simulink model "gm_pmsm_decoder_slrt"  (R2020b)
settings: Solver=FixedStepDiscrete  StartTime=0.0  StopTime=20  FixedStep=Ts  RelTol=1e-3
PostLoadFcn:
  | try
  | cell = struct2cell(dir(fullfile(speedgoatroot_hdlb, 'hdlsrc', 'pwm', '*.vhd')));
  | addSourceFiles = strjoin(fullfile(cell(2,:),cell(1,:)), ';');
  | hdlset_param('pwm_example_hdlc/DUT PWM and CAP', 'IPCoreAdditionalFiles', addSourceFiles);
  | end
InitFcn:
  | Ts=50e-6;     % Simulation time step
  | kp = 1e6;   % Proportional gain
  | ki =1e2;   % Integral gain
  | fsw = 5e3;     % Switching frequency
  | Vdc = 400;     % Inverter DC supply voltage
  | Rs = 0.1;     % Stator resistance
  | Ld = 2e-3;   % Inductance (d axis)
  | Lq = 2e-3;   % Inductance (q axis)
  | PM = 0.28;        % Flux linkage
  | N = 1;               % Pole pairs
undefined symbols (not defined in the file): Copy_of_gm_pmsm_fpga_pcie_slrt, DiscIntNeverNeededParam, FPGA, IO334
libraries: speedgoatlib_hdlCoder_IO3xx x19, powerlib x9, powerlib_meascontrol x4, eeGeneralControl x3, quadrature_cpulib x2, mcbcontrolslib x1, slrealtimeutilitieslib x1, pwm_cpulib x1, mcbplantlib x1
settings Model: ModifiedByFormat=Speedgoat GmbH  SimulationMode=external  Creator=Speedgoat GmbH  LastModifiedBy=Speedgoat GmbH
settings SolverCC: ConcurrentTasks=on  PositivePriorityOrder=on
settings DataIOCC: LimitDataPoints=on  SaveFormat=Array  ReturnWorkspaceOutputs=off
settings OptimizationCC: BlockReduction=off  ConditionallyExecuteInputs=off  DefaultParameterBehavior=Inlined  OptimizeBlockIOStorage=off
settings DebuggingCC: AlgebraicLoopMsg=error  UnderspecifiedInitializationDetection=Classic  MergeDetectMultiDrivingBlocksExec=none  SolverPrmCheckMsg=warning  InheritedTsInSrcMsg=none  SingleTaskRateTransMsg=error  TasksWithSamePriorityMsg=none  ParameterPrecisionLossMsg=none  PregeneratedLibrarySubsystemCodeDiagnostic=none  SFUnexpectedBacktrackingDiag=warning  SFNoUnconditionalDefaultTransitionDiag=warning  SFExecutionAtInitializationDiag=none  ArithmeticOperatorsInVariantConditions=warning
settings HardwareCC: ProdBitPerLong=64  ProdLongLongMode=on  ProdHWDeviceType=Intel->x86-64 (Linux 64)  TargetBitPerPointer=64  TargetBitPerSizeT=64  TargetBitPerPtrDiffT=64  TargetLongLongMode=on  TargetIntDivRoundTo=Zero  TargetEndianess=LittleEndian  TargetWordSize=64  TargetHWDeviceType=Custom Processor->MATLAB Host Computer
settings ModelReferenceCC: PropagateSignalLabelsOutOfModel=off
settings SFSimCC: SimUseLocalCustomCode=off  CustomCodeUndefinedFunction=UseInterfaceOnly
settings RTWCC: Description=Simulink Real-Time  SystemTargetFile=slrealtime.tlc  TemplateMakefile=slrealtime_default_tmf  RTWUseLocalCustomCode=off  Toolchain=Simulink Real-Time Toolchain  BuildConfiguration=Faster Runs  CodeExecutionProfiling=on  TargetLang=C++
settings CodeAppCC: StateflowObjectComments=on
settings ConfigComp: CovMetricSettings=dw  CovSaveCumulativeToWorkspaceVar=on  CovSaveSingleToWorkspaceVar=on  CovExternalEMLEnable=off

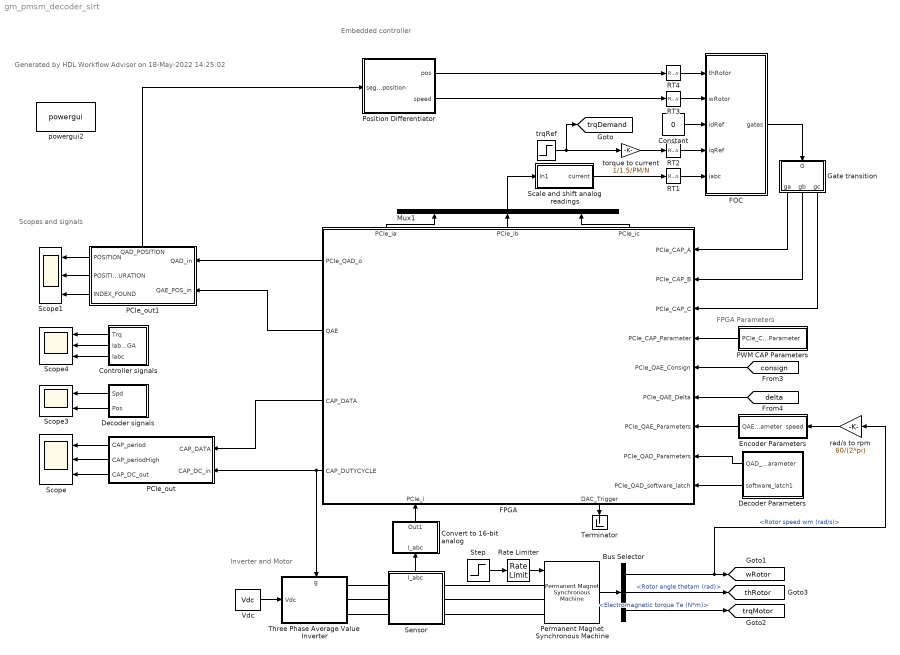
== system gm_pmsm_decoder_slrt ==
  note: Inverter and Motor
  note: FPGA Parameters
  note: Embedded controller
  note: Scopes and signals
  note: Generated by HDL Workflow Advisor on 18-May-2022 14:25:02
  Bus Selector : BusSelector  OutputSignals=Rotor speed wm (rad/s),Rotor angle thetam (rad),Electromagnetic torque Te (N*m)
  Constant : Constant  Value=0  SampleTime=-1
  Controller signals : Subsystem
  Convert to 16-bit analog : Subsystem
  Decoder Parameters : Subsystem
  Decoder signals : Subsystem
  Encoder Parameters : Subsystem
  FOC : Subsystem
  FPGA : Subsystem  mask(Speedgoat IO334-325k Interface Block){module_id=1, slot=-1, ts=-1, FpgaFreq=100}
      mask prompts: module_id "FPGA Module Identifier:"; slot "PCI slot (-1: autosearch):"; ts "Sample time:"; FpgaFreq "FPGA Frequency [MHz]"
      mask help: Simulink Real-Time Interface Block for Speedgoat IO334-325k.
      mask init:
      | hdlslrt.backend.mfpgaparameters;
      settings: PortSchema="{\"entries\":[{\"content\":{\"sides\":[{\"content\":{\"connectorIds\":[\"Out5\",\"Out6\",\"Out7\",\"Out8\"]},\"type\":\"ConnectorPlacement.EquallySpacedRectSide\",\"uuid\":\"34ddc533-e92e-4f84-ab54-56ee31c34ed5\"},{\"content\":{\"connectorIds\":[\"In2\",\"In3\",\"In4\",\"In5\",\"In6\",\"In7\",\"In8\",\"In9\",\"In10\"],\"side\":\"RIGHT\"},\"type\":\"ConnectorPlacement.EquallySpacedRectSide\",\"uuid\":\"fc43732f-8b85-47c9-af73-b87840a05fb5\"},{\"content\":{\"connectorIds\":[\"Out2\",\"Out3\",\"Out4\"],\"side\":\"TOP\"},\"type\":\"ConnectorPlacement.EquallySpacedRectSide\",\"uuid\":\"bf663b9c-33b6-4726-afdb-56df835214b8\"},{\"content\":{\"connectorIds\":[\"In1\",\"Out1\"],\"side\":\"BOTTOM\"},\"type\":\"ConnectorPlacement.EquallySpacedRectSide\",\"uuid\":\"04fbffa8-14ef-4425-a219-a420a37a7cbf\"},{\"content\":{\"connectorIds\":[],\"side\":\"HIDDEN\"},\"type\":\"ConnectorPlacement.EquallySpacedRectSide\",\"uuid\":\"ed9b2637-afe7-435a-b994-99eac90c9c32\"}]},\"type\":\"ConnectorPlacement.EquallySpacedConnector\",\"uuid\":\"b4b9272a-3f4d-4e79-a573-4a3ad4933ba9\"}],\"packageUris\":[\"http://schema.mathworks.com/mf0/Connector/R2020b\"],\"version\":\"1.0\"}"
      mask Help: eval('speedgoatdoc_hdlc')
      mask Display:
      | SetupBlkPath = find_system(gcb, 'LookUnderMasks', 'all', 'FollowLinks', 'on', 'regexp', 'on', 'Name', 'IO3(\d|x){2}\s+Setup' );
      | SetupBlkPath = SetupBlkPath{1};
      | TS = get_param(SetupBlkPath,'timestamp_mcs');
      | disp(sprintf('Speedgoat IO334-325k\nFPGA I/O Module\n\nTimestamp\n%s\n\nReference Design\nVersion 2.1\n\nMatlab R2020b\n\nPCIe Link Width: X4\nRear Plugin: -21\nAurora Mode: None\nAurora Byteswap: true\n', TS))
  Gate transition : Subsystem
  Mux1 : Mux  Inputs=3
  PCIe_out : Subsystem
  PCIe_out1 : Subsystem
      settings: PortSchema="{\"entries\":[{\"content\":{\"sides\":[{\"content\":{\"connectorIds\":[\"In1\",\"In2\"]},\"type\":\"ConnectorPlacement.EquallySpacedRectSide\",\"uuid\":\"af69b108-ebc1-4eba-857b-579d7c2071b1\"},{\"content\":{\"connectorIds\":[\"Out1\",\"Out2\",\"Out3\"],\"side\":\"RIGHT\"},\"type\":\"ConnectorPlacement.EquallySpacedRectSide\",\"uuid\":\"109121c9-5293-4b78-b0df-8505743611a0\"},{\"content\":{\"connectorIds\":[\"Out4\"],\"side\":\"TOP\"},\"type\":\"ConnectorPlacement.EquallySpacedRectSide\",\"uuid\":\"7680958f-0bbc-4169-a54e-ff3c19fd2e64\"},{\"content\":{\"connectorIds\":[],\"side\":\"HIDDEN\"},\"type\":\"ConnectorPlacement.EquallySpacedRectSide\",\"uuid\":\"af8ad87e-ac41-49e8-9442-a6b24975ced8\"}]},\"type\":\"ConnectorPlacement.EquallySpacedConnector\",\"uuid\":\"27b07649-0e95-47d8-9bc5-7790ead06fb5\"}],\"packageUris\":[\"http://schema.mathworks.com/mf0/Connector/R2020b\"],\"version\":\"1.0\"}"
  PWM CAP Parameters : Subsystem
  Permanent Magnet Synchronous Machine : powerlib/Machines/Permanent Magnet Synchronous Machine  NbPhases=3  FluxDistribution=Sinusoidal  RotorType=Salient-pole  MechanicalLoad=Speed w  PresetModel=No  ShowDetailedParameters=on  MeasurementBus=off  Resistance=Rs  Inductance=8.5e-3  dqInductances=[Ld Lq]  La=0.000395  MachineConstant=Flux linkage established by magnets (V.s)  Flux=PM  VoltageCst=50.7864  TorqueCst=0.42  Flat=120  Mechanical=[0.0027 0.0004924 1 0]  PolePairs=N  InitialConditions=[0,0, 0,0]  InitialConditions5ph=[0 0 0 0 0 0]  RefAngle=Aligned with phase A axis (original Park)  IterativeDiscreteModel=Trapezoidal non iterative  TsBlock=-1  TsPowergui=0
  Position Differentiator : Subsystem
  RT{1..4} (4 alike) : RateTransition  OutPortSampleTimeOpt=Inherit  OutPortSampleTime=Ts
  Rate Limiter : RateLimiter  RisingSlewLimit=100/60*2*pi  SampleTimeMode=inherited
  Scale and shift analog readings : Subsystem
  Scope : Scope  NumInputPorts=3
  Scope1 : Scope  NumInputPorts=3
  Scope3 : Scope  NumInputPorts=2
  Scope4 : Scope  NumInputPorts=3
  Sensor : Subsystem
      settings: PortSchema="{\"entries\":[{\"content\":{\"sides\":[{\"content\":{\"connectorIds\":[\"LConn1\",\"LConn2\",\"LConn3\"]},\"type\":\"ConnectorPlacement.EquallySpacedRectSide\",\"uuid\":\"d3673cf9-f798-4f95-832a-0ee38b3b4235\"},{\"content\":{\"connectorIds\":[\"RConn1\",\"RConn2\",\"RConn3\"],\"side\":\"RIGHT\"},\"type\":\"ConnectorPlacement.EquallySpacedRectSide\",\"uuid\":\"f1c3e6c7-7356-4e8b-bcca-414f2c82a0be\"},{\"content\":{\"connectorIds\":[\"Out1\"],\"side\":\"TOP\"},\"type\":\"ConnectorPlacement.EquallySpacedRectSide\",\"uuid\":\"10e31bf8-a182-46d8-beca-1ec9bb9081e0\"},{\"content\":{\"connectorIds\":[],\"side\":\"HIDDEN\"},\"type\":\"ConnectorPlacement.EquallySpacedRectSide\",\"uuid\":\"21150a95-24d3-4ba1-92b8-5619804d049c\"}]},\"type\":\"ConnectorPlacement.EquallySpacedConnector\",\"uuid\":\"db0d9e3c-2d98-4024-a8e1-7fc9e86b9a02\"}],\"packageUris\":[\"http://schema.mathworks.com/mf0/Connector/R2020b\"],\"version\":\"1.0\"}"
  Step : Step  Time=0.01  After=500/60*2*pi  SampleTime=0
  Terminator : Terminator
  Three Phase Average Value Inverter : Subsystem
      settings: PortSchema="{\"entries\":[{\"content\":{\"sides\":[{\"content\":{\"connectorIds\":[\"In1\"]},\"type\":\"ConnectorPlacement.EquallySpacedRectSide\",\"uuid\":\"bfacb710-2d3a-4e7b-9063-25c8b87226b9\"},{\"content\":{\"connectorIds\":[\"RConn1\",\"RConn2\",\"RConn3\"],\"side\":\"RIGHT\"},\"type\":\"ConnectorPlacement.EquallySpacedRectSide\",\"uuid\":\"a8d38f79-eb95-4afe-ba2f-2842c1cba801\"},{\"content\":{\"connectorIds\":[\"In2\"],\"side\":\"TOP\"},\"type\":\"ConnectorPlacement.EquallySpacedRectSide\",\"uuid\":\"291d9d52-08e6-4456-8afe-095013b7df64\"},{\"content\":{\"connectorIds\":[],\"side\":\"HIDDEN\"},\"type\":\"ConnectorPlacement.EquallySpacedRectSide\",\"uuid\":\"61aa80b0-9b99-474b-ab67-e014373e5595\"}]},\"type\":\"ConnectorPlacement.EquallySpacedConnector\",\"uuid\":\"1232c420-125a-43af-99e1-be04cd6c95a4\"}],\"packageUris\":[\"http://schema.mathworks.com/mf0/Connector/R2020b\"],\"version\":\"1.0\"}"
  Vdc : Constant  Value=Vdc  SampleTime=Ts
  powergui2 : powerlib/powergui  Priority=1  SimulationMode=Discrete  SampleTime=Ts  frequency=60  Iterations=50  frequencyindice=0  Pbase=100e6  ErrMax=1e-4  UnitsV=kV  UnitsW=MW  buscounter=0  FunctionMessages=off  echomessages=off  EnableUseOfTLC=off  CurrentSourceSwitches=off  DisableSnubberDevices=off  DisableRonSwitches=off  DisableVfSwitches=off  DisplayEquations=off  AutomaticDiscreteSolvers=off  SolverType=Tustin/Backward Euler (TBE)  Interpol=off  ExternalGateDelay=off  methode=off  Ts=100  x0status=blocks  SPID=on  SwTol=0  HookPort=off  NonlinearTolerance=1e-4  nMaxIteration=100  ContinueOnMaxIteration=off  RestoreLinks=warning  ResistiveCurrentMeasurement=off  Frange=[0:2:500]  Ylog=off  Xlog=on  ShowGrid=off  save=off  variable=ZData  structure=0  ZoomFFT=off  StartTime=0.0  cycles=1  DisplayStyle=1  fundamental=60  FreqAxis=off  MaxFrequency=1000  frequencyindicesteady=1  RmsSteady=1  display=off
  rad/s to rpm : Gain  Gain=60/(2*pi)
  torque to current : Gain  Gain=1/1.5/PM/N  SaturateOnIntegerOverflow=on  OutDataTypeStr=Inherit: Same as input  ParamDataTypeStr=Inherit: Same as input
  trqRef : Step  Time=0.3  After=300  SampleTime=Ts
  tag scope: thRotor=global, trqDemand=global, trqMotor=global, wRotor=global
  wires:
  Convert to 16-bit analog/1(Out1) -> FPGA/1(PCIe_i)
  Decoder Parameters/2(software_latch1) -> FPGA/10(PCIe_QAD_software_latch)
  Decoder Parameters/1(QAD_parameter) -> FPGA/9(PCIe_QAD_Parameters)
  FPGA/5(PCIe_QAD_o) -> PCIe_out1/1(QAD_in)
  PCIe_out1/2(POSITION_DURATION) -> Scope1/2
  PCIe_out1/3(INDEX_FOUND) -> Scope1/3
  PCIe_out1/1(POSITION) -> Scope1/1
  RT4/1 -> FOC/1(thRotor)
  Controller signals/3(Iabc) -> Scope4/3
  Controller signals/2(Iabc_FPGA) -> Scope4/2
  Controller signals/1(Trq) -> Scope4/1
  Rate Limiter/1 -> Permanent Magnet Synchronous Machine/1
  Vdc/1 -> Three Phase Average Value Inverter/1(Vdc)
  Bus Selector/2 -> [thRotor]  "<Rotor angle thetam (rad)>"
  FPGA/8(CAP_DUTYCYCLE) -> Three Phase Average Value Inverter/2(g), PCIe_out/2(CAP_DC_in)
  Sensor/1(I_abc) -> Convert to 16-bit analog/1(I_abc)
  Bus Selector/1 -> [wRotor], rad/s to rpm/1  "<Rotor speed wm (rad/s)>"
  Permanent Magnet Synchronous Machine/1 -> Bus Selector/1
  Bus Selector/3 -> [trqMotor]  "<Electromagnetic torque Te (N*m)>"
  FOC/1(gates) -> Gate transition/1(G)
  Constant/1 -> FOC/3(idRef)
  torque to current/1 -> RT2/1
  PCIe_out/3(CAP_DC_out) -> Scope/3
  PCIe_out/2(CAP_periodHigh) -> Scope/2
  PCIe_out/1(CAP_period) -> Scope/1
  Encoder Parameters/1(QAE_parameter) -> FPGA/8(PCIe_QAE_Parameters)
  PWM CAP Parameters/1(PCIe_CAP_Parameter) -> FPGA/5(PCIe_CAP_Parameter)
  FPGA/7(CAP_DATA) -> PCIe_out/1(CAP_DATA)
  rad/s to rpm/1 -> Encoder Parameters/1(speed)
  FPGA/6(QAE) -> PCIe_out1/2(QAE_POS_in)
  RT3/1 -> FOC/2(wRotor)
  RT2/1 -> FOC/4(iqRef)
  RT1/1 -> FOC/5(iabc)
  trqRef/1 -> torque to current/1, [trqDemand]
  FPGA/3(PCIe_ib) -> Mux1/2
  FPGA/2(PCIe_ia) -> Mux1/1
  FPGA/4(PCIe_ic) -> Mux1/3
  FPGA/1(DAC_Trigger) -> Terminator/1
  Decoder signals/1(Spd) -> Scope3/1
  Decoder signals/2(Pos) -> Scope3/2
  [delta] -> FPGA/7(PCIe_QAE_Delta)
  [consign] -> FPGA/6(PCIe_QAE_Consign)
  Gate transition/1(ga) -> FPGA/2(PCIe_CAP_A)
  Gate transition/2(gb) -> FPGA/3(PCIe_CAP_B)
  Gate transition/3(gc) -> FPGA/4(PCIe_CAP_C)
  Mux1/1 -> Scale and shift analog readings/1(In1)
  Scale and shift analog readings/1(current) -> RT1/1
  Step/1 -> Rate Limiter/1
  PCIe_out1/4(QAD_POSITION) -> Position Differentiator/1(segment position)
  Position Differentiator/1(pos) -> RT4/1
  Position Differentiator/2(speed) -> RT3/1
  connections:
  Permanent Magnet Synchronous Machine/LConn2 -- Sensor/RConn2
  Permanent Magnet Synchronous Machine/LConn3 -- Sensor/RConn3
  Sensor/LConn3 -- Three Phase Average Value Inverter/RConn3
  Sensor/LConn1 -- Three Phase Average Value Inverter/RConn1
  Sensor/LConn2 -- Three Phase Average Value Inverter/RConn2
  Permanent Magnet Synchronous Machine/LConn1 -- Sensor/RConn1

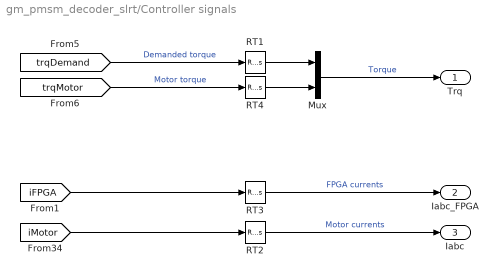
== system gm_pmsm_decoder_slrt/Controller signals ==
  Mux : Mux  Inputs=2
  RT{1..4} (4 alike) : RateTransition  OutPortSampleTime=Ts
  Trq : Outport  VectorParamsAs1DForOutWhenUnconnected=off
  Iabc_FPGA : Outport  Port=2  VectorParamsAs1DForOutWhenUnconnected=off
  Iabc : Outport  Port=3  VectorParamsAs1DForOutWhenUnconnected=off
  wires:
  [trqDemand] -> RT1/1  "Demanded torque"
  RT1/1 -> Mux/1
  RT3/1 -> Iabc_FPGA/1  "FPGA currents"
  [iMotor] -> RT2/1
  RT2/1 -> Iabc/1  "Motor currents"
  [iFPGA] -> RT3/1
  Mux/1 -> Trq/1  "Torque"
  [trqMotor] -> RT4/1  "Motor torque"
  RT4/1 -> Mux/2

== system gm_pmsm_decoder_slrt/Convert to 16-bit analog ==
  I_abc : Inport
  1-D Lookup Table : Lookup_n-D  NumberOfTableDimensions=1  BreakpointsForDimension1=[-2^15, 2^15-1]  Table=[0, 3.3/10*(2^15-1)]  ExtrapMethod=Clip  InternalRulePriority=Speed  RndMeth=Simplest  InputSameDT=on
  Data Type Conversion : DataTypeConversion  OutDataTypeStr=int16
  Gain : Gain  Gain=2^3
  Out1 : Outport
  wires:
  Data Type Conversion/1 -> Out1/1
  1-D Lookup Table/1 -> Data Type Conversion/1
  I_abc/1 -> Gain/1
  Gain/1 -> 1-D Lookup Table/1

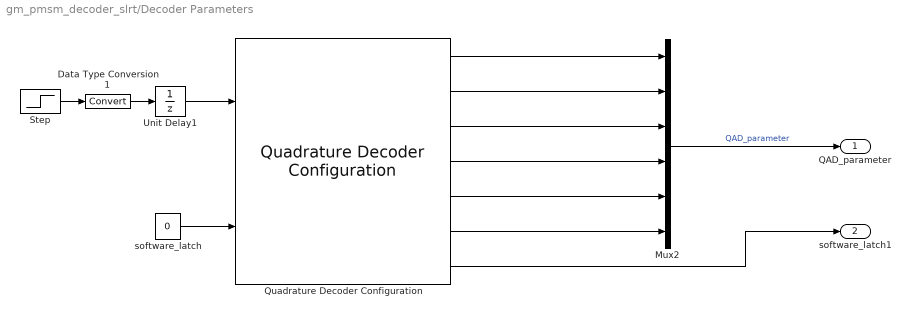
== system gm_pmsm_decoder_slrt/Decoder Parameters ==
  Data Type Conversion1 : DataTypeConversion
  Mux2 : Mux  Inputs=6
  Quadrature Decoder Configuration : quadrature_cpulib/Quadrature Decoder Configuration  FPGA_freq=100e6  n_channels=1  samplingMode=2x  indexControlMode=Reset on index  latchMode=Continuous  lowerLimit=0  upperLimit=512
      settings: SourceProductName=Simulink Real-Time: Speedgoat HDL Blockset
  Step : Step  Time=0.002
  Unit Delay1 : UnitDelay  SampleTime=-1  HasFrameUpgradeWarning=on
  software_latch : Constant  Value=0  SampleTime=-1
  QAD_parameter : Outport
  software_latch1 : Outport  Port=2
  wires:
  Quadrature Decoder Configuration/7 -> software_latch1/1
  Mux2/1 -> QAD_parameter/1  "QAD_parameter"
  software_latch/1 -> Quadrature Decoder Configuration/2
  Quadrature Decoder Configuration/1 -> Mux2/1
  Quadrature Decoder Configuration/6 -> Mux2/6
  Quadrature Decoder Configuration/4 -> Mux2/4
  Quadrature Decoder Configuration/3 -> Mux2/3
  Data Type Conversion1/1 -> Unit Delay1/1
  Quadrature Decoder Configuration/5 -> Mux2/5
  Step/1 -> Data Type Conversion1/1
  Unit Delay1/1 -> Quadrature Decoder Configuration/1
  Quadrature Decoder Configuration/2 -> Mux2/2

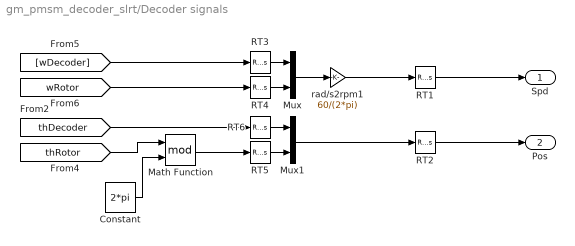
== system gm_pmsm_decoder_slrt/Decoder signals ==
  Constant : Constant  Value=2*pi  SampleTime=-1
  Math Function : Math  Operator=mod  SaturateOnIntegerOverflow=on
  Mux : Mux  Inputs=2
  Mux1 : Mux  Inputs=2
  RT{1..6} (6 alike) : RateTransition  OutPortSampleTime=Ts
  rad/s2rpm1 : Gain  Gain=60/(2*pi)
  Spd : Outport  VectorParamsAs1DForOutWhenUnconnected=off
  Pos : Outport  Port=2  VectorParamsAs1DForOutWhenUnconnected=off
  wires:
  [wDecoder] -> RT3/1
  Mux/1 -> rad/s2rpm1/1
  Mux1/1 -> RT2/1
  [wRotor] -> RT4/1
  RT1/1 -> Spd/1
  RT2/1 -> Pos/1
  RT4/1 -> Mux/2
  RT5/1 -> Mux1/2
  rad/s2rpm1/1 -> RT1/1
  RT3/1 -> Mux/1
  RT6/1 -> Mux1/1
  [thDecoder] -> RT6/1
  Constant/1 -> Math Function/2
  [thRotor] -> Math Function/1
  Math Function/1 -> RT5/1

== system gm_pmsm_decoder_slrt/Encoder Parameters ==
  speed : Inport
  Mux2 : Mux  Inputs=7
  Quadrature Encoder Configuration : quadrature_cpulib/Quadrature Encoder Configuration  fpgaFreq=100e6  n_channels=1  numSeg=[512]  phaseAngle=90  initPos=[0]  freeWheel=on
      settings: SourceProductName=Simulink Real-Time: Speedgoat HDL Blockset
  Step : Step  Time=0.002
  position : Constant  Value=8  SampleTime=-1
  QAE_parameter : Outport
  tag scope: consign=global, delta=global
  wires:
  speed/1 -> Quadrature Encoder Configuration/3
  Quadrature Encoder Configuration/8 -> [consign]
  Step/1 -> Quadrature Encoder Configuration/1
  Quadrature Encoder Configuration/7 -> Mux2/7
  Quadrature Encoder Configuration/4 -> Mux2/4
  Quadrature Encoder Configuration/2 -> Mux2/2
  position/1 -> Quadrature Encoder Configuration/2
  Mux2/1 -> QAE_parameter/1  "QAE_parameter"
  Quadrature Encoder Configuration/6 -> Mux2/6
  Quadrature Encoder Configuration/5 -> Mux2/5
  Quadrature Encoder Configuration/1 -> Mux2/1  "position"
  Quadrature Encoder Configuration/9 -> [delta]
  Quadrature Encoder Configuration/3 -> Mux2/3

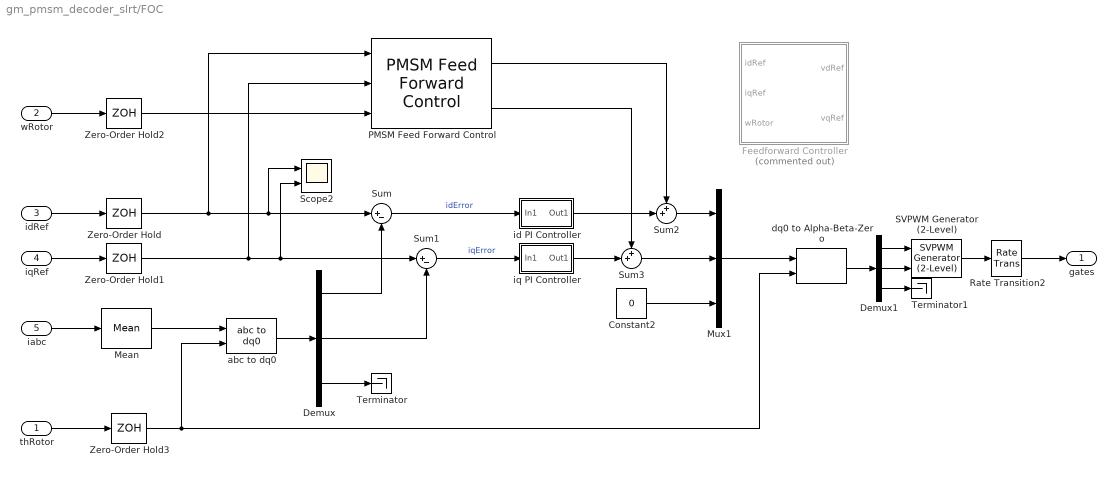
== system gm_pmsm_decoder_slrt/FOC ==
  thRotor : Inport
  wRotor : Inport  Port=2
  idRef : Inport  Port=3
  iqRef : Inport  Port=4
  iabc : Inport  Port=5
  Constant2 : Constant  Value=0  SampleTime=-1
  Demux : Demux  Outputs=3
  Demux1 : Demux  Outputs=3
  Feedforward Controller : Subsystem  Commented=on
  Mean : powerlib_meascontrol/Measurements/Mean  Freq=fsw  Vinit=0  Ts=Ts
  Mux1 : Mux  Inputs=3
  PMSM Feed Forward Control : mcbcontrolslib/PMSM Feed Forward Control  polePairs=N  Ld=Ld  Lq=Lq  FluxPM=PM  V_dc=Vdc/sqrt(3)  Units=SI Units  V_base=24/sqrt(3)  I_base=19.3  N_base=4107
      settings: SourceProductBaseCode=MT
  Rate Transition2 : RateTransition
  SVPWM Generator (2-Level) : powerlib_meascontrol/Pulse & Signal Generators/SVPWM Generator (2-Level)  InputType=alpha-beta components  SwitchingPattern=Pattern #1  Fc=fsw  ParUref=[0.8 -30 50]  Ts=Ts
      settings: SourceProductBaseCode=PS
  Scope2 : Scope  NumInputPorts=2
  Sum : Sum  Inputs=|+-
  Sum1 : Sum  Inputs=|+-
  Sum2 : Sum  Inputs=++|
  Sum3 : Sum  Inputs=++|
  Terminator : Terminator
  Terminator1 : Terminator
  Zero-Order Hold{,1..3} (4 alike) : ZeroOrderHold  SampleTime=-1
  abc to dq0 : powerlib_meascontrol/Transformations/abc to dq0  Alignment=Aligned with phase A axis
  dq0 to Alpha-Beta-Zero : powerlib_meascontrol/Transformations/dq0 to Alpha-Beta-Zero  Alignment=Aligned with phase A axis
      settings: SourceProductBaseCode=PS
  id PI Controller : Subsystem
  iq PI Controller : Subsystem
  gates : Outport  VectorParamsAs1DForOutWhenUnconnected=off
  wires:
  Zero-Order Hold3/1 -> dq0 to Alpha-Beta-Zero/2, abc to dq0/2
  Zero-Order Hold2/1 -> PMSM Feed Forward Control/3
  iqRef/1 -> Zero-Order Hold1/1
  idRef/1 -> Zero-Order Hold/1
  PMSM Feed Forward Control/2 -> Sum3/1
  PMSM Feed Forward Control/1 -> Sum2/1
  Constant2/1 -> Mux1/3
  Demux/1 -> Sum/2
  dq0 to Alpha-Beta-Zero/1 -> Demux1/1
  Demux1/2 -> SVPWM Generator (2-Level)/2
  SVPWM Generator (2-Level)/1 -> Rate Transition2/1
  id PI Controller/1(Out1) -> Sum2/2
  Sum2/1 -> Mux1/1
  Sum3/1 -> Mux1/2
  Demux/2 -> Sum1/2
  Sum1/1 -> iq PI Controller/1(In1)  "iqError"
  iabc/1 -> Mean/1
  Demux1/3 -> Terminator1/1
  Mux1/1 -> dq0 to Alpha-Beta-Zero/1
  Mean/1 -> abc to dq0/1
  wRotor/1 -> Zero-Order Hold2/1
  thRotor/1 -> Zero-Order Hold3/1
  Rate Transition2/1 -> gates/1
  Zero-Order Hold1/1 -> Scope2/2, Sum1/1, PMSM Feed Forward Control/2
  abc to dq0/1 -> Demux/1
  Sum/1 -> id PI Controller/1(In1)  "idError"
  Demux1/1 -> SVPWM Generator (2-Level)/1
  Zero-Order Hold/1 -> Sum/1, Scope2/1, PMSM Feed Forward Control/1
  iq PI Controller/1(Out1) -> Sum3/2
  Demux/3 -> Terminator/1

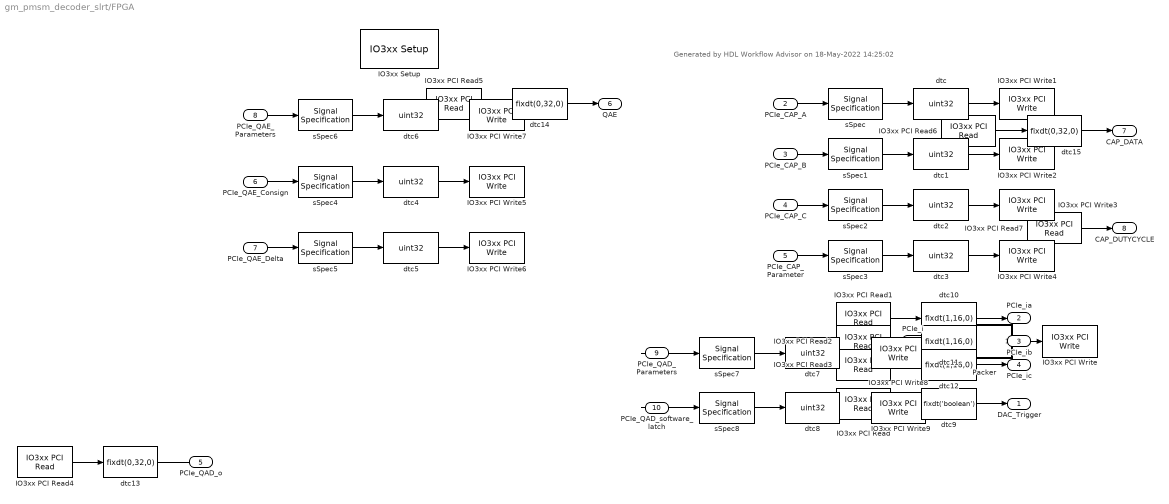
== system gm_pmsm_decoder_slrt/FPGA ==
  note: Generated by HDL Workflow Advisor on 18-May-2022 14:25:02
  PCIe_i : Inport  OutDataTypeStr=int16
  PCIe_CAP_A : Inport  Port=2
  PCIe_CAP_B : Inport  Port=3
  PCIe_CAP_C : Inport  Port=4
  PCIe_CAP_Parameter : Inport  Port=5
  PCIe_QAE_Consign : Inport  Port=6
  PCIe_QAE_Delta : Inport  Port=7
  PCIe_QAE_Parameters : Inport  Port=8
  PCIe_QAD_Parameters : Inport  Port=9
  PCIe_QAD_software_latch : Inport  Port=10
  IO3xx PCI Read : speedgoatlib_hdlCoder_IO3xx/IO3xx PCI Read  device_id=1  module_id=module_id  board_type=IO334-325k  port_name=DAC_Trigger  port_offset=hex2dec('134')  port_type=uint32  port_dim=1  strobe=0  sample_time=ts
  IO3xx PCI Read1 : speedgoatlib_hdlCoder_IO3xx/IO3xx PCI Read  device_id=1  module_id=module_id  board_type=IO334-325k  port_name=PCIe_ia  port_offset=hex2dec('138')  port_type=uint32  port_dim=1  strobe=0  sample_time=ts
  IO3xx PCI Read2 : speedgoatlib_hdlCoder_IO3xx/IO3xx PCI Read  device_id=1  module_id=module_id  board_type=IO334-325k  port_name=PCIe_ib  port_offset=hex2dec('13C')  port_type=uint32  port_dim=1  strobe=0  sample_time=ts
  IO3xx PCI Read3 : speedgoatlib_hdlCoder_IO3xx/IO3xx PCI Read  device_id=1  module_id=module_id  board_type=IO334-325k  port_name=PCIe_ic  port_offset=hex2dec('144')  port_type=uint32  port_dim=1  strobe=0  sample_time=ts
  IO3xx PCI Read4 : speedgoatlib_hdlCoder_IO3xx/IO3xx PCI Read  device_id=1  module_id=module_id  board_type=IO334-325k  port_name=PCIe_QAD_o  port_offset=hex2dec('1D0')  port_type=uint32  port_dim=4  strobe=hex2dec('1E0')  sample_time=ts
  IO3xx PCI Read5 : speedgoatlib_hdlCoder_IO3xx/IO3xx PCI Read  device_id=1  module_id=module_id  board_type=IO334-325k  port_name=QAE  port_offset=hex2dec('150')  port_type=uint32  port_dim=1  strobe=0  sample_time=ts
  IO3xx PCI Read6 : speedgoatlib_hdlCoder_IO3xx/IO3xx PCI Read  device_id=1  module_id=module_id  board_type=IO334-325k  port_name=CAP_DATA  port_offset=hex2dec('200')  port_type=uint32  port_dim=18  strobe=hex2dec('280')  sample_time=ts
  IO3xx PCI Read7 : speedgoatlib_hdlCoder_IO3xx/IO3xx PCI Read  device_id=1  module_id=module_id  board_type=IO334-325k  port_name=CAP_DUTYCYCLE  port_offset=hex2dec('290')  port_type=single  port_dim=3  strobe=hex2dec('2A0')  sample_time=ts
  IO3xx PCI Write : speedgoatlib_hdlCoder_IO3xx/IO3xx PCI Write  device_id=1  module_id=module_id  board_type=IO334-325k  port_name=PCIe_i  port_offset=hex2dec('100')  port_type=uint32  port_dim=2  strobe=hex2dec('108')  sample_time=ts
  IO3xx PCI Write1 : speedgoatlib_hdlCoder_IO3xx/IO3xx PCI Write  device_id=1  module_id=module_id  board_type=IO334-325k  port_name=PCIe_CAP_A  port_offset=hex2dec('10C')  port_type=uint32  port_dim=1  strobe=0  sample_time=ts
  IO3xx PCI Write2 : speedgoatlib_hdlCoder_IO3xx/IO3xx PCI Write  device_id=1  module_id=module_id  board_type=IO334-325k  port_name=PCIe_CAP_B  port_offset=hex2dec('110')  port_type=uint32  port_dim=1  strobe=0  sample_time=ts
  IO3xx PCI Write3 : speedgoatlib_hdlCoder_IO3xx/IO3xx PCI Write  device_id=1  module_id=module_id  board_type=IO334-325k  port_name=PCIe_CAP_C  port_offset=hex2dec('114')  port_type=uint32  port_dim=1  strobe=0  sample_time=ts
  IO3xx PCI Write4 : speedgoatlib_hdlCoder_IO3xx/IO3xx PCI Write  device_id=1  module_id=module_id  board_type=IO334-325k  port_name=PCIe_CAP_Parameter  port_offset=hex2dec('120')  port_type=uint32  port_dim=3  strobe=hex2dec('130')  sample_time=ts
  IO3xx PCI Write5 : speedgoatlib_hdlCoder_IO3xx/IO3xx PCI Write  device_id=1  module_id=module_id  board_type=IO334-325k  port_name=PCIe_QAE_Consign  port_offset=hex2dec('140')  port_type=uint32  port_dim=1  strobe=0  sample_time=ts
  IO3xx PCI Write6 : speedgoatlib_hdlCoder_IO3xx/IO3xx PCI Write  device_id=1  module_id=module_id  board_type=IO334-325k  port_name=PCIe_QAE_Delta  port_offset=hex2dec('118')  port_type=uint32  port_dim=1  strobe=0  sample_time=ts
  IO3xx PCI Write7 : speedgoatlib_hdlCoder_IO3xx/IO3xx PCI Write  device_id=1  module_id=module_id  board_type=IO334-325k  port_name=PCIe_QAE_Parameters  port_offset=hex2dec('160')  port_type=uint32  port_dim=7  strobe=hex2dec('180')  sample_time=ts
  IO3xx PCI Write8 : speedgoatlib_hdlCoder_IO3xx/IO3xx PCI Write  device_id=1  module_id=module_id  board_type=IO334-325k  port_name=PCIe_QAD_Parameters  port_offset=hex2dec('1A0')  port_type=uint32  port_dim=6  strobe=hex2dec('1C0')  sample_time=ts
  IO3xx PCI Write9 : speedgoatlib_hdlCoder_IO3xx/IO3xx PCI Write  device_id=1  module_id=module_id  board_type=IO334-325k  port_name=PCIe_QAD_software_latch  port_offset=hex2dec('11C')  port_type=uint32  port_dim=1  strobe=0  sample_time=ts
  IO3xx Setup : speedgoatlib_hdlCoder_IO3xx/IO3xx Setup  mdl_ss_name=Copy_of_gm_pmsm_fpga_pcie_slrt/FPGA  board_type=IO334-325k  fpga_sync_mode=on  reset_mode=on  device_id=1  module_id=module_id  pci_slot=slot  fpga_mat_file=hdl_prj\hdlsrc\Copy_of_gm_pmsm_fpga_pcie_slrt\FPGA.mat  timestamp_mcs=05/18/22 14:10:29  timestamp=2205181323  tsreg=hex2dec('8')  bsf_file=FPGA_2205181323.mcs  mcs=0
  Packer : Subsystem
  dtc{,1..8} (9 alike) : DataTypeConversion  OutDataTypeStr=uint32  ConvertRealWorld=Stored Integer (SI)  RndMeth=Zero
  dtc10 : DataTypeConversion  OutDataTypeStr=fixdt(1,16,0)  ConvertRealWorld=Stored Integer (SI)  RndMeth=Zero
  dtc11 : DataTypeConversion  OutDataTypeStr=fixdt(1,16,0)  ConvertRealWorld=Stored Integer (SI)  RndMeth=Zero
  dtc12 : DataTypeConversion  OutDataTypeStr=fixdt(1,16,0)  ConvertRealWorld=Stored Integer (SI)  RndMeth=Zero
  dtc13 : DataTypeConversion  OutDataTypeStr=fixdt(0,32,0)  ConvertRealWorld=Stored Integer (SI)  RndMeth=Zero
  dtc14 : DataTypeConversion  OutDataTypeStr=fixdt(0,32,0)  ConvertRealWorld=Stored Integer (SI)  RndMeth=Zero
  dtc15 : DataTypeConversion  OutDataTypeStr=fixdt(0,32,0)  ConvertRealWorld=Stored Integer (SI)  RndMeth=Zero
  dtc9 : DataTypeConversion  OutDataTypeStr=fixdt('boolean')  ConvertRealWorld=Stored Integer (SI)  RndMeth=Zero
  sSpec{,1..2,8} (4 alike) : SignalSpecification  OutDataTypeStr=fixdt('boolean')
  sSpec3 : SignalSpecification  OutDataTypeStr=fixdt(0,32,0)
  sSpec4 : SignalSpecification  OutDataTypeStr=fixdt(0,32,0)
  sSpec5 : SignalSpecification  OutDataTypeStr=fixdt(1,32,0)
  sSpec6 : SignalSpecification  OutDataTypeStr=fixdt(0,32,0)
  sSpec7 : SignalSpecification  OutDataTypeStr=fixdt(1,32,0)
  DAC_Trigger : Outport
  PCIe_ia : Outport  Port=2
  PCIe_ib : Outport  Port=3
  PCIe_ic : Outport  Port=4
  PCIe_QAD_o : Outport  Port=5  VectorParamsAs1DForOutWhenUnconnected=off
  QAE : Outport  Port=6
  CAP_DATA : Outport  Port=7
  CAP_DUTYCYCLE : Outport  Port=8
  wires:
  PCIe_i/1 -> Packer/1(unpacked)
  Packer/1(packed) -> IO3xx PCI Write/1
  PCIe_CAP_A/1 -> sSpec/1
  sSpec/1 -> dtc/1
  dtc/1 -> IO3xx PCI Write1/1
  PCIe_CAP_B/1 -> sSpec1/1
  sSpec1/1 -> dtc1/1
  dtc1/1 -> IO3xx PCI Write2/1
  PCIe_CAP_C/1 -> sSpec2/1
  sSpec2/1 -> dtc2/1
  dtc2/1 -> IO3xx PCI Write3/1
  PCIe_CAP_Parameter/1 -> sSpec3/1
  sSpec3/1 -> dtc3/1
  dtc3/1 -> IO3xx PCI Write4/1
  PCIe_QAE_Consign/1 -> sSpec4/1
  sSpec4/1 -> dtc4/1
  dtc4/1 -> IO3xx PCI Write5/1
  PCIe_QAE_Delta/1 -> sSpec5/1
  sSpec5/1 -> dtc5/1
  dtc5/1 -> IO3xx PCI Write6/1
  PCIe_QAE_Parameters/1 -> sSpec6/1
  sSpec6/1 -> dtc6/1
  dtc6/1 -> IO3xx PCI Write7/1
  PCIe_QAD_Parameters/1 -> sSpec7/1
  sSpec7/1 -> dtc7/1
  dtc7/1 -> IO3xx PCI Write8/1
  PCIe_QAD_software_latch/1 -> sSpec8/1
  sSpec8/1 -> dtc8/1
  dtc8/1 -> IO3xx PCI Write9/1
  dtc9/1 -> DAC_Trigger/1
  IO3xx PCI Read/1 -> dtc9/1
  dtc10/1 -> PCIe_ia/1
  IO3xx PCI Read1/1 -> dtc10/1
  dtc11/1 -> PCIe_ib/1
  IO3xx PCI Read2/1 -> dtc11/1
  dtc12/1 -> PCIe_ic/1
  IO3xx PCI Read3/1 -> dtc12/1
  dtc13/1 -> PCIe_QAD_o/1
  IO3xx PCI Read4/1 -> dtc13/1
  dtc14/1 -> QAE/1
  IO3xx PCI Read5/1 -> dtc14/1
  dtc15/1 -> CAP_DATA/1
  IO3xx PCI Read6/1 -> dtc15/1
  IO3xx PCI Read7/1 -> CAP_DUTYCYCLE/1

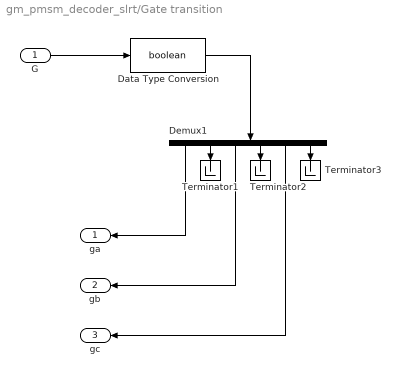
== system gm_pmsm_decoder_slrt/Gate transition ==
  G : Inport
  Data Type Conversion : DataTypeConversion  OutDataTypeStr=boolean
  Demux1 : Demux  Outputs=6
  Terminator1 : Terminator
  Terminator2 : Terminator
  Terminator3 : Terminator
  ga : Outport
  gb : Outport  Port=2
  gc : Outport  Port=3
  wires:
  Data Type Conversion/1 -> Demux1/1
  Demux1/2 -> Terminator1/1
  Demux1/6 -> Terminator3/1
  G/1 -> Data Type Conversion/1
  Demux1/4 -> Terminator2/1
  Demux1/1 -> ga/1
  Demux1/3 -> gb/1
  Demux1/5 -> gc/1

== system gm_pmsm_decoder_slrt/PCIe_out ==
  CAP_DATA : Inport
  CAP_DC_in : Inport  Port=2
  Bus Creator : BusCreator  Inputs=6
  Bus Selector : BusSelector  OutputSignals=PCIe_CAP_Period,PCIe_CAP_periodHigh
  Demux : Demux  Outputs=6
  CAP_period : Outport
  CAP_periodHigh : Outport  Port=2
  CAP_DC_out : Outport  Port=3
  wires:
  CAP_DC_in/1 -> CAP_DC_out/1  "CAP_DutyCycle"
  Bus Selector/2 -> CAP_periodHigh/1  "<PCIe_CAP_periodHigh>"
  Bus Selector/1 -> CAP_period/1  "<PCIe_CAP_Period>"
  Demux/6 -> Bus Creator/6  "PCIe_CAP_Data_Valid"
  Demux/3 -> Bus Creator/3  "PCIe_CAP_periodLow"
  Demux/2 -> Bus Creator/2  "PCIe_CAP_periodHigh"
  Demux/4 -> Bus Creator/4  "PCIe_CAP_TOn"
  Bus Creator/1 -> Bus Selector/1
  Demux/1 -> Bus Creator/1  "PCIe_CAP_Period"
  Demux/5 -> Bus Creator/5  "PCIe_CAP_TOff"
  CAP_DATA/1 -> Demux/1

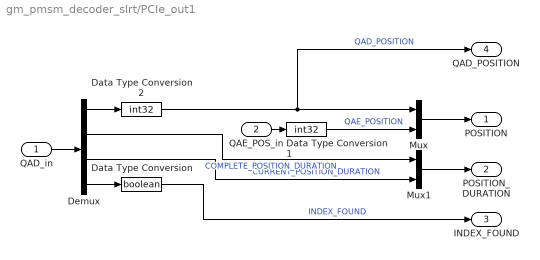
== system gm_pmsm_decoder_slrt/PCIe_out1 ==
  QAD_in : Inport
  QAE_POS_in : Inport  Port=2
  Data Type Conversion : DataTypeConversion  OutDataTypeStr=boolean
  Data Type Conversion1 : DataTypeConversion  OutDataTypeStr=int32
  Data Type Conversion2 : DataTypeConversion  OutDataTypeStr=int32
  Demux : Demux
  Mux : Mux  Inputs=2
  Mux1 : Mux  Inputs=2
  POSITION : Outport
  POSITION_DURATION : Outport  Port=2
  INDEX_FOUND : Outport  Port=3
  QAD_POSITION : Outport  Port=4
  wires:
  QAE_POS_in/1 -> Data Type Conversion1/1
  Demux/1 -> Data Type Conversion2/1
  Data Type Conversion/1 -> INDEX_FOUND/1  "INDEX_FOUND"
  Demux/4 -> Data Type Conversion/1
  Data Type Conversion2/1 -> Mux/1, QAD_POSITION/1  "QAD_POSITION"
  Demux/3 -> Mux1/2  "CURRENT_POSITION_DURATION"
  QAD_in/1 -> Demux/1
  Demux/2 -> Mux1/1  "COMPLETE_POSITION_DURATION"
  Mux/1 -> POSITION/1
  Mux1/1 -> POSITION_DURATION/1
  Data Type Conversion1/1 -> Mux/2  "QAE_POSITION"

== system gm_pmsm_decoder_slrt/PWM CAP Parameters ==
  Data Type Conversion4 : DataTypeConversion  OutDataTypeStr=uint32
  Data Type Conversion5 : DataTypeConversion  OutDataTypeStr=uint32
  Data Type Conversion6 : DataTypeConversion  OutDataTypeStr=uint32
  Mux1 : Mux  Inputs=3
  PWM Capture Configuration : pwm_cpulib/PWM Capture Configuration  FPGA_freq=100e6  n_channels=1  captureMode=High transitions triggered  captureTimeout=0  PWM_pattern_en=off
      settings: SourceProductName=Simulink Real-Time: Speedgoat HDL Blockset
  PCIe_CAP_Parameter : Outport
  wires:
  PWM Capture Configuration/2 -> Data Type Conversion5/1
  Data Type Conversion6/1 -> Mux1/3
  Data Type Conversion5/1 -> Mux1/2
  Data Type Conversion4/1 -> Mux1/1
  PWM Capture Configuration/3 -> Data Type Conversion6/1
  Mux1/1 -> PCIe_CAP_Parameter/1
  PWM Capture Configuration/1 -> Data Type Conversion4/1

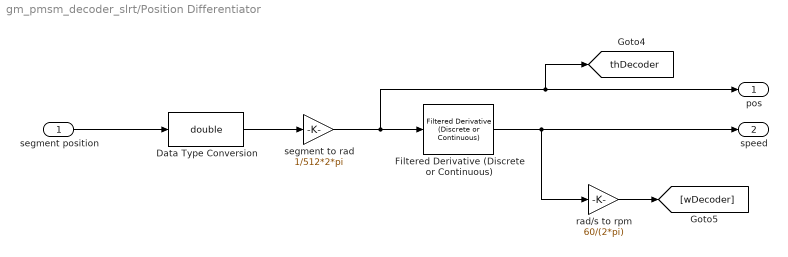
== system gm_pmsm_decoder_slrt/Position Differentiator ==
  segment position : Inport
  Data Type Conversion : DataTypeConversion  OutDataTypeStr=double
  Filtered Derivative (Discrete or Continuous) : eeGeneralControl/Filtered Derivative (Discrete or Continuous)  K=1  T=0.001  B=inf  A=-inf  minRatio=10  init_option=Specify as parameter  x0=0  Ts=-1
      settings: SourceProductBaseCode=PS
  rad/s to rpm : Gain  Gain=60/(2*pi)
  segment to rad : Gain  Gain=1/512*2*pi
  pos : Outport
  speed : Outport  Port=2
  tag scope: thDecoder=global
  wires:
  segment position/1 -> Data Type Conversion/1
  Filtered Derivative (Discrete or Continuous)/1 -> rad/s to rpm/1, speed/1
  segment to rad/1 -> pos/1, [thDecoder], Filtered Derivative (Discrete or Continuous)/1
  Data Type Conversion/1 -> segment to rad/1
  rad/s to rpm/1 -> [wDecoder]

== system gm_pmsm_decoder_slrt/Scale and shift analog readings ==
  In1 : Inport
  1-D Lookup Table : Lookup_n-D  NumberOfTableDimensions=1  BreakpointsForDimension1=[0, 3.3/10*(2^15-1)]  Table=[-2^15, 2^15-1]  ExtrapMethod=Clip  InternalRulePriority=Speed  RndMeth=Simplest  InputSameDT=on
  Data Type Conversion : DataTypeConversion  OutDataTypeStr=double
  Scale to max range : Gain  Gain=2^-3
  current : Outport
  tag scope: iFPGA=global
  wires:
  Data Type Conversion/1 -> 1-D Lookup Table/1
  1-D Lookup Table/1 -> Scale to max range/1
  In1/1 -> Data Type Conversion/1
  Scale to max range/1 -> current/1, [iFPGA]  "current"

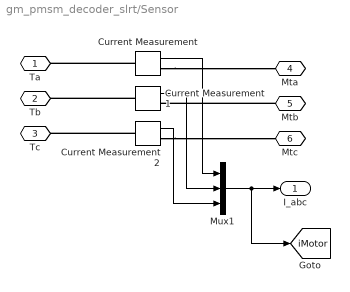
== system gm_pmsm_decoder_slrt/Sensor ==
  Current Measurement : powerlib/Measurements/Current Measurement  PhasorSimulation=off  OutputType=Complex  PSBequivalent=0
  Current Measurement1 : powerlib/Measurements/Current Measurement  PhasorSimulation=off  OutputType=Complex  PSBequivalent=0
  Current Measurement2 : powerlib/Measurements/Current Measurement  PhasorSimulation=off  OutputType=Complex  PSBequivalent=0
  Mux1 : Mux  Inputs=3
  Ta : PMIOPort  Side=Left
  Tb : PMIOPort  Port=2  Side=Left
  Tc : PMIOPort  Port=3  Side=Left
  Mta : PMIOPort  Port=4  Side=Right
  Mtb : PMIOPort  Port=5  Side=Right
  Mtc : PMIOPort  Port=6  Side=Right
  I_abc : Outport  VectorParamsAs1DForOutWhenUnconnected=off
  tag scope: iMotor=global
  wires:
  Mux1/1 -> I_abc/1, [iMotor]
  Current Measurement2/1 -> Mux1/3
  Current Measurement/1 -> Mux1/1
  Current Measurement1/1 -> Mux1/2
  connections:
  Current Measurement2/RConn1 -- Mtc/RConn1
  Current Measurement2/LConn1 -- Tc/RConn1
  Current Measurement/LConn1 -- Ta/RConn1
  Current Measurement/RConn1 -- Mta/RConn1
  Current Measurement1/LConn1 -- Tb/RConn1
  Mtb/RConn1 -- Current Measurement1/RConn1

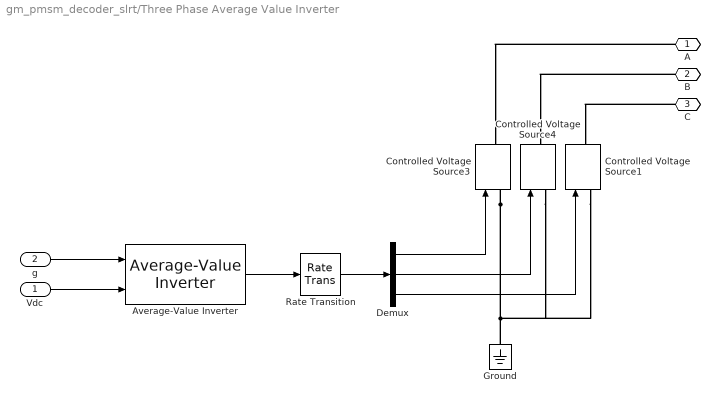
== system gm_pmsm_decoder_slrt/Three Phase Average Value Inverter ==
  Vdc : Inport
  g : Inport  Port=2
  Average-Value Inverter : mcbplantlib/Average-Value Inverter
  Controlled Voltage Source1 : powerlib/Electrical Sources/Controlled Voltage Source  Initialize=on  Source_Type=AC  Amplitude=0  Phase=0  Frequency=0  Measurements=None
  Controlled Voltage Source3 : powerlib/Electrical Sources/Controlled Voltage Source  Initialize=on  Source_Type=AC  Amplitude=0  Phase=0  Frequency=0  Measurements=None
  Controlled Voltage Source4 : powerlib/Electrical Sources/Controlled Voltage Source  Initialize=on  Source_Type=AC  Amplitude=0  Phase=0  Frequency=0  Measurements=None
  Demux : Demux  Outputs=3
  Ground : powerlib/Elements/Ground  LConnTagsString=a
  Rate Transition : RateTransition
  A : PMIOPort  Tag=PMCPort  Side=Right
  B : PMIOPort  Tag=PMCPort  Port=2  Side=Right
  C : PMIOPort  Tag=PMCPort  Port=3  Side=Right
  wires:
  Demux/3 -> Controlled Voltage Source1/1
  Vdc/1 -> Average-Value Inverter/2
  Demux/2 -> Controlled Voltage Source4/1
  Demux/1 -> Controlled Voltage Source3/1
  g/1 -> Average-Value Inverter/1
  Rate Transition/1 -> Demux/1
  Average-Value Inverter/1 -> Rate Transition/1
  connections:
  A/RConn1 -- Controlled Voltage Source3/RConn1
  B/RConn1 -- Controlled Voltage Source4/RConn1
  C/RConn1 -- Controlled Voltage Source1/RConn1
  Controlled Voltage Source3/LConn1 -- Controlled Voltage Source4/LConn1 -- Controlled Voltage Source1/LConn1 -- Ground/LConn1

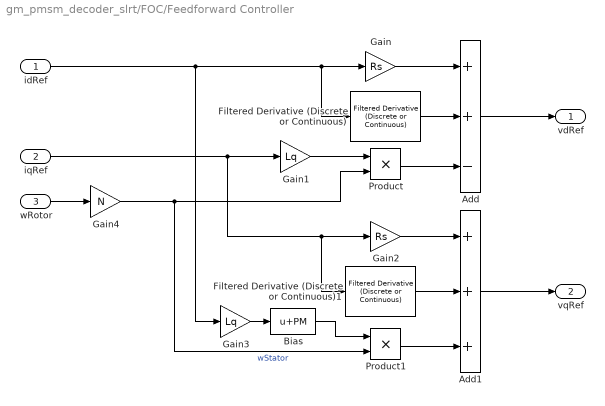
== system gm_pmsm_decoder_slrt/FOC/Feedforward Controller ==
  idRef : Inport
  iqRef : Inport  Port=2
  wRotor : Inport  Port=3
  Add : Sum  Inputs=++-
  Add1 : Sum  Inputs=+++
  Bias : Bias  Bias=PM  SaturateOnIntegerOverflow=on
  Filtered Derivative (Discrete or Continuous) : eeGeneralControl/Filtered Derivative (Discrete or Continuous)  K=Ld  T=1e-3  B=inf  A=-inf  minRatio=10  init_option=Specify as parameter  x0=0  Ts=-1
      settings: SourceProductBaseCode=PS
  Filtered Derivative (Discrete or Continuous)1 : eeGeneralControl/Filtered Derivative (Discrete or Continuous)  K=Lq  T=1e-3  B=inf  A=-inf  minRatio=10  init_option=Specify as parameter  x0=0  Ts=-1
      settings: SourceProductBaseCode=PS
  Gain : Gain  Gain=Rs
  Gain1 : Gain  Gain=Lq
  Gain2 : Gain  Gain=Rs
  Gain3 : Gain  Gain=Lq
  Gain4 : Gain  Gain=N
  Product : Product
  Product1 : Product
  vdRef : Outport
  vqRef : Outport  Port=2
  wires:
  Add1/1 -> vqRef/1
  Gain3/1 -> Bias/1
  Product/1 -> Add/3
  Bias/1 -> Product1/1
  Filtered Derivative (Discrete or Continuous)1/1 -> Add1/2
  iqRef/1 -> Gain1/1, Filtered Derivative (Discrete or Continuous)1/1, Gain2/1
  Filtered Derivative (Discrete or Continuous)/1 -> Add/2
  Gain2/1 -> Add1/1
  Product1/1 -> Add1/3
  Gain1/1 -> Product/1
  idRef/1 -> Gain/1, Filtered Derivative (Discrete or Continuous)/1, Gain3/1
  Gain/1 -> Add/1
  Gain4/1 -> Product1/2, Product/2  "wStator"
  Add/1 -> vdRef/1
  wRotor/1 -> Gain4/1

== system gm_pmsm_decoder_slrt/FOC/id PI Controller ==
  In1 : Inport
  Discrete-Time Integrator : DiscreteIntegrator  gainval=ki  SampleTime=-1  LimitOutput=on  UpperSaturationLimit=1  LowerSaturationLimit=-1  ICPrevOutput=DiscIntNeverNeededParam  ICPrevScaledInput=DiscIntNeverNeededParam
  Gain2 : Gain  Gain=kp  SaturateOnIntegerOverflow=on  OutDataTypeStr=Inherit: Same as input  ParamDataTypeStr=Inherit: Same as input
  Sum2 : Sum  Inputs=++|
  Out1 : Outport  VectorParamsAs1DForOutWhenUnconnected=off
  wires:
  Discrete-Time Integrator/1 -> Sum2/1
  Sum2/1 -> Out1/1
  In1/1 -> Gain2/1, Discrete-Time Integrator/1
  Gain2/1 -> Sum2/2

== system gm_pmsm_decoder_slrt/FOC/iq PI Controller ==
  In1 : Inport
  Discrete-Time Integrator : DiscreteIntegrator  gainval=ki  SampleTime=-1  LimitOutput=on  UpperSaturationLimit=1  LowerSaturationLimit=-1  ICPrevOutput=DiscIntNeverNeededParam  ICPrevScaledInput=DiscIntNeverNeededParam
  Gain2 : Gain  Gain=kp  SaturateOnIntegerOverflow=on  OutDataTypeStr=Inherit: Same as input  ParamDataTypeStr=Inherit: Same as input
  Sum2 : Sum  Inputs=++|
  Out1 : Outport  VectorParamsAs1DForOutWhenUnconnected=off
  wires:
  Discrete-Time Integrator/1 -> Sum2/1
  Sum2/1 -> Out1/1
  In1/1 -> Gain2/1, Discrete-Time Integrator/1
  Gain2/1 -> Sum2/2

== system gm_pmsm_decoder_slrt/FPGA/Packer ==
  unpacked : Inport
  pack : slrealtimeutilitieslib/Bit Packing  MaskBitPatterns={[0:15 16:31 32:47 ]}  MaskPackDataType=uint32  MaskPackDataSize=2
      settings: SourceProductBaseCode=XP
  sSpec : SignalSpecification  OutDataTypeStr=fixdt(1,16,0)
  upconvert : DataTypeConversion  OutDataTypeStr=uint16  ConvertRealWorld=Stored Integer (SI)  RndMeth=Zero
  packed : Outport
  wires:
  unpacked/1 -> sSpec/1
  sSpec/1 -> upconvert/1
  upconvert/1 -> pack/1
  pack/1 -> packed/1
